simulink model "TAU_PID_Controller"  (R2017a)
settings: Solver=VariableStepAuto  StartTime=0.0  StopTime=100  RelTol=1e-3
libraries: dspnetwork x3
settings Model: Creator=Андрей  LastModifiedBy=Андрей

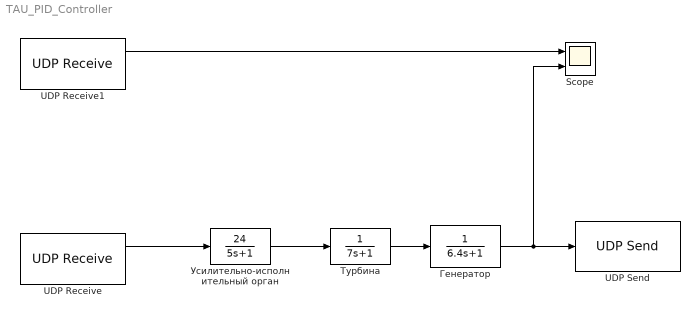
== system TAU_PID_Controller ==
  Scope : Scope  NumInputPorts=2
  UDP Receive : dspnetwork/UDP Receive  localURL='0.0.0.0'  localPort=9101  remoteURL='localhost'  remotePort=-1  recvBufferSize=8192  dims=1  signalDatatype=double  isVarSize=off  showBlockingTime=off  blockingTime=0  sampletime=1  blockPlatform=[]
  UDP Receive1 : dspnetwork/UDP Receive  localURL='0.0.0.0'  localPort=9111  remoteURL='localhost'  remotePort=-1  recvBufferSize=8192  dims=1  signalDatatype=double  isVarSize=off  showBlockingTime=off  blockingTime=0  sampletime=0.001  blockPlatform=[]
  UDP Send : dspnetwork/UDP Send  remoteURL='localhost'  remotePort=9031  localURL='0.0.0.0'  localPortSource=Automatically determine  localPort=-1  sampletime=-1  blockPlatform=[]  separateLengthPort=0
  Генератор : TransferFcn  Denominator=[6.4 1]
  Турбина : TransferFcn  Denominator=[7 1]
  Усилительно-исполнительный орган : TransferFcn  Numerator=[24]  Denominator=[5 1]
  wires:
  Усилительно-исполнительный орган/1 -> Турбина/1
  Генератор/1 -> Scope/2, UDP Send/1
  Турбина/1 -> Генератор/1
  UDP Receive/1 -> Усилительно-исполнительный орган/1
  UDP Receive1/1 -> Scope/1
